simulink model "AltControlSimulink_4_16_17"  (R2016a)
settings: Solver=VariableStepAuto  StartTime=0.0  StopTime=7200  RelTol=1e-3
settings Model: Creator=alexismitchnick  LastModifiedBy=alexismitchnick
settings SolverCC: SolverJacobianMethodControl=FullAnalytical  ZeroCrossControl=DisableAll

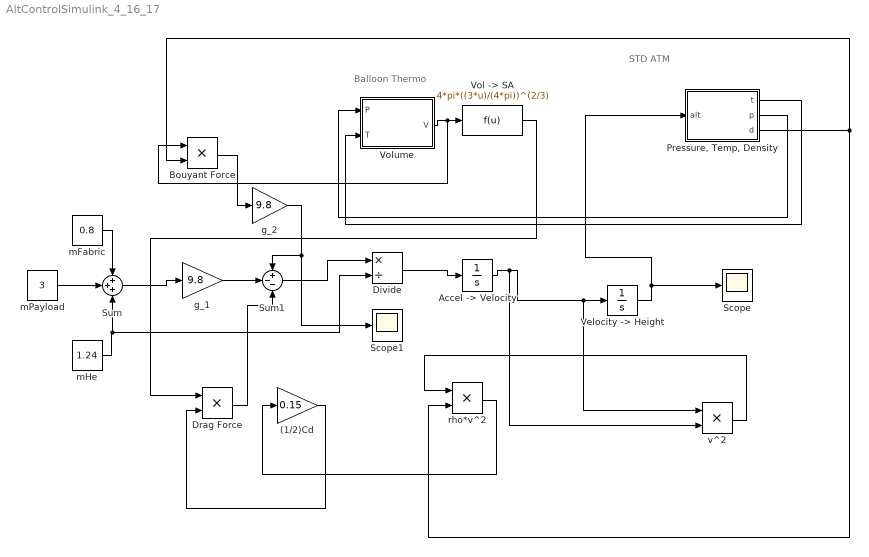
== system AltControlSimulink_4_16_17 ==
  note: Balloon Thermo
  note: STD ATM
  (1/2)Cd : Gain  Gain=0.15
  "Accel -> Velocity" : Integrator
  Bouyant Force : Product
  Divide : Product  Inputs=*/
  Drag Force : Product
  "Pressure, Temp, Density" : MATLAB Function  TreatAsAtomicUnit=on
  Scope : Scope
  Scope1 : Scope
  Sum : Sum  Inputs=+++
  Sum1 : Sum  Inputs=+--
  "Velocity -> Height" : Integrator
  "Vol -> SA" : Fcn  Expr=4*pi*((3*u)/(4*pi))^(2/3)
  Volume : MATLAB Function  TreatAsAtomicUnit=on
  "g_1 " : Gain  Gain=9.8
  g_2 : Gain  Gain=9.8
  mFabric : Constant  Value=0.8
  mHe : Constant  Value=1.24
  mPayload : Constant  Value=3
  rho*v^2 : Product
  v^2 : Product
  wires:
  mFabric/1 -> Sum/1
  mPayload/1 -> Sum/2
  Sum/1 -> "g_1 "/1
  "g_1 "/1 -> Sum1/2
  mHe/1 -> Divide/2, Sum/3
  Sum1/1 -> Divide/1
  Divide/1 -> "Accel -> Velocity"/1
  "Accel -> Velocity"/1 -> v^2/2, v^2/1, "Velocity -> Height"/1
  Drag Force/1 -> Sum1/3
  "Pressure, Temp, Density"/3(d) -> Bouyant Force/2, rho*v^2/2
  "Vol -> SA"/1 -> Drag Force/1
  v^2/1 -> rho*v^2/1
  rho*v^2/1 -> (1/2)Cd/1
  (1/2)Cd/1 -> Drag Force/2
  Bouyant Force/1 -> g_2/1
  "Velocity -> Height"/1 -> "Pressure, Temp, Density"/1(alt), Scope/1
  Volume/1(V) -> Bouyant Force/1, "Vol -> SA"/1
  g_2/1 -> Sum1/1, Scope1/1
  "Pressure, Temp, Density"/2(p) -> Volume/1(P)
  "Pressure, Temp, Density"/1(t) -> Volume/2(T)

== matlab function AltControlSimulink_4_16_17/Pressure, Temp, Density ==
  data: alt input; t output; p output; d output
function [t,p,d] = getTPD(alt)
    if alt <= 11000
        t = 15.04 - 0.00649*alt;
        p = 101.29 * ((t + 273.1)/288.08)^5.256;
    elseif (11000 < alt) && (alt <= 25000)
        t = -56.46;
        p = 22.65 * exp(1.73 - 0.000157*alt);
    else
        t = -131.21 + 0.00299*alt;
        p = 2.488 * ((t + 273.1)/216.6)^(-11.38);
    end
    d = p/(0.2869 * (t + 273.1));
end

== matlab function AltControlSimulink_4_16_17/Volume ==
  data: P input; V output; T input
function V = fcn(P,T)
mHe = 1.24;
R = 2.0769;

V = (mHe*R*(T+273))/P;
